simulink model "ThreePhaseThyristorRectifier"  (R2018b)
settings: Solver=FixedStepDiscrete  StartTime=0.0  StopTime=0.04  FixedStep=1e-8  RelTol=1e-3
libraries: powerlib x13
settings Model: Creator=Sam  LastModifiedBy=Sam

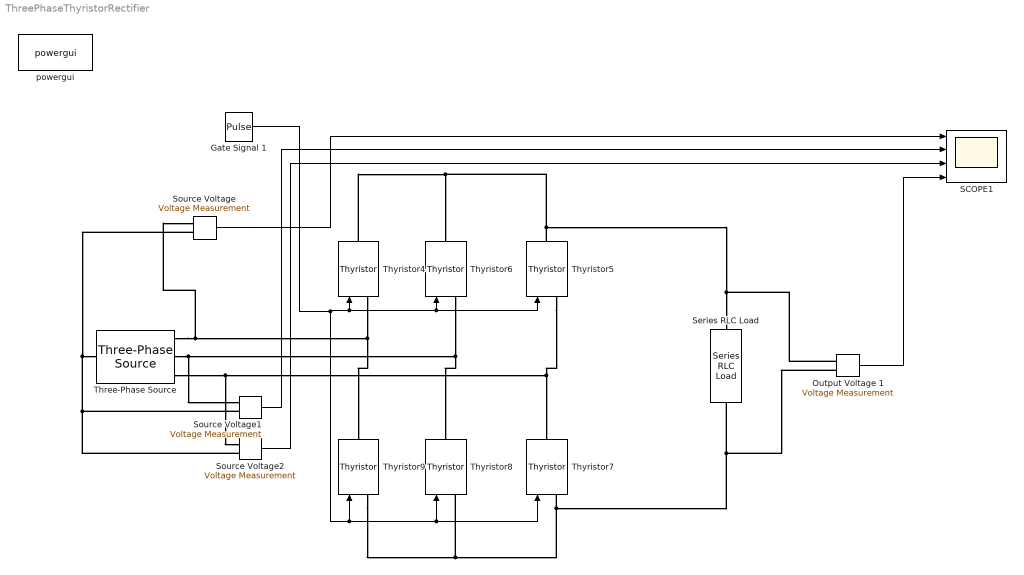
== system ThreePhaseThyristorRectifier ==
  Gate Signal 1 : DiscretePulseGenerator  PulseType=Time based  Amplitude=20  Period=3.333e-3  PulseWidth=5  PhaseDelay=3.333e-3
  Output Voltage 1 : powerlib/Measurements/Voltage Measurement  PhasorSimulation=off  OutputType=Complex  PSBequivalent=0
  SCOPE1 : Scope  NumInputPorts=4
  Series RLC Load : powerlib/Elements/Series RLC Load  LConnTagsString=a  RConnTagsString=__new0  NominalVoltage=230  NominalFrequency=50  ActivePower=1600  InductivePower=0  CapacitivePower=0  Setx0=off  InitialVoltage=0  SetiL0=off  InitialCurrent=0  Measurements=None  LoadType=constant Z
  Source Voltage : powerlib/Measurements/Voltage Measurement  PhasorSimulation=off  OutputType=Complex  PSBequivalent=0
  Source Voltage1 : powerlib/Measurements/Voltage Measurement  PhasorSimulation=off  OutputType=Complex  PSBequivalent=0
  Source Voltage2 : powerlib/Measurements/Voltage Measurement  PhasorSimulation=off  OutputType=Complex  PSBequivalent=0
  Three-Phase Source : powerlib/Electrical Sources/Three-Phase Source  InternalConnection=Yn  VoltagePhases=off  Voltage=398.37  PhaseAngle=0  Voltage_phases=[25e3 25e3 25e3]/sqrt(3)  PhaseAngles_phases=[0 -120 +120]  Frequency=50  NonIdealSource=off  SpecifyImpedance=off  Resistance=0.00001  Inductance=16.58e-3  ShortCircuitLevel=100e6  BaseVoltage=25e3  XRratio=7  BusType=swing  Pref=10e3  Qref=0  Prefabc=[10e3, 10e3, 10e3]  Qrefabc=[0, 0, 0]  Qmin=-inf  Qmax=inf
  Thyristor{4..9} (6 alike) : powerlib/Power Electronics/Thyristor  Ron=0.00001  Lon=0  Vf=0  IC=0  Rs=1e5  Cs=inf  Measurements=off
  powergui : powerlib/powergui  Priority=1  SimulationMode=Discrete  SampleTime=1e-8  frequency=60  Iterations=50  frequencyindice=50  Pbase=100e6  ErrMax=1e-4  UnitsV=kV  UnitsW=MW  buscounter=0  FunctionMessages=off  echomessages=off  EnableUseOfTLC=off  CurrentSourceSwitches=off  DisableSnubberDevices=off  DisableRonSwitches=off  DisableVfSwitches=off  DisplayEquations=off  SolverType=Tustin/Backward Euler (TBE)  Interpol=off  ExternalGateDelay=off  methode=off  Ts=100  x0status=blocks  SPID=on  SwTol=0  HookPort=off  RestoreLinks=warning  ResistiveCurrentMeasurement=off  Frange=[0:2:500]  Ylog=off  Xlog=on  ShowGrid=off  save=off  variable=ZData  structure=0  ZoomFFT=off  StartTime=0.0  cycles=1  DisplayStyle=1  fundamental=60  FreqAxis=off  MaxFrequency=1000  frequencyindicesteady=1  RmsSteady=1  display=off
  wires:
  Gate Signal 1/1 -> Thyristor5/1, Thyristor6/1, Thyristor4/1, Thyristor8/1, Thyristor7/1, Thyristor9/1
  Output Voltage 1/1 -> SCOPE1/4
  Source Voltage/1 -> SCOPE1/1
  Source Voltage1/1 -> SCOPE1/2
  Source Voltage2/1 -> SCOPE1/3
  connections:
  Thyristor5/LConn1 -- Source Voltage2/LConn1 -- Three-Phase Source/RConn3 -- Thyristor7/RConn1
  Thyristor6/LConn1 -- Three-Phase Source/RConn2 -- Source Voltage1/LConn1 -- Thyristor8/RConn1
  Thyristor4/LConn1 -- Three-Phase Source/RConn1 -- Source Voltage/LConn1 -- Thyristor9/RConn1
  Thyristor4/RConn1 -- Output Voltage 1/LConn1 -- Series RLC Load/LConn1 -- Thyristor5/RConn1 -- Thyristor6/RConn1
  Thyristor9/LConn1 -- Output Voltage 1/LConn2 -- Series RLC Load/RConn1 -- Thyristor7/LConn1 -- Thyristor8/LConn1
  Source Voltage/LConn2 -- Source Voltage1/LConn2 -- Source Voltage2/LConn2 -- Three-Phase Source/LConn1
